simulink model "HandlerSOMANET"  (R2016b)
settings: Solver=VariableStepAuto  StartTime=0.0  StopTime=10.0  RelTol=1e-3
settings Model: DataDictionary=ModelDictionary.sldd  Creator=Nathan  LastModifiedBy=Nathan

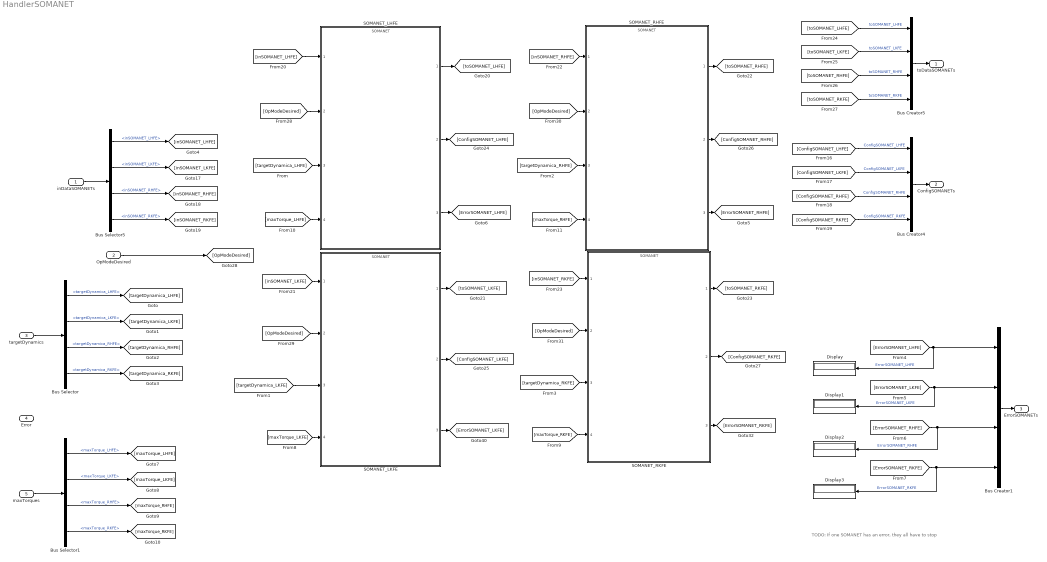
== system HandlerSOMANET ==
  note: TODO: If one SOMANET has an error, they all have to stop
  inDataSOMANETs : Inport  OutDataTypeStr=Bus: inDataSOMANETs  BusOutputAsStruct=on
  OpModeDesired : Inport  Port=2
  targetDynamics : Inport  Port=3  OutDataTypeStr=Bus: targetDynamics  BusOutputAsStruct=on
  Error : Inport  Port=4  BusOutputAsStruct=on
  maxTorques : Inport  Port=5  OutDataTypeStr=Bus: maxTorques  BusOutputAsStruct=on
  Bus Creator1 : BusCreator  Inputs=4  OutDataTypeStr=Bus: toSafetySOMANETs  NonVirtualBus=on
  Bus Creator4 : BusCreator  Inputs=4  OutDataTypeStr=Bus: ConfigSOMANETs  NonVirtualBus=on
  Bus Creator5 : BusCreator  Inputs=4
  Bus Selector : BusSelector  OutputSignals=targetDynamica_LHFE,targetDynamica_LKFE,targetDynamica_RHFE,targetDynamica_RKFE
  Bus Selector1 : BusSelector  OutputSignals=maxTorque_LHFE,maxTorque_LKFE,maxTorque_RHFE,maxTorque_RKFE
  Bus Selector5 : BusSelector  OutputSignals=inSOMANET_LHFE,inSOMANET_LKFE,inSOMANET_RHFE,inSOMANET_RKFE
  Display{,1..3} (4 alike) : Display
  SOMANET_LHFE : ModelReference  ModelNameDialog=SOMANET.slx  SimulationMode=Normal  ModelReferenceVersion=1.37
  SOMANET_LKFE : ModelReference  ModelNameDialog=SOMANET.slx  SimulationMode=Normal  ModelReferenceVersion=1.37
  SOMANET_RHFE : ModelReference  ModelNameDialog=SOMANET.slx  SimulationMode=Normal  ModelReferenceVersion=1.37
  SOMANET_RKFE : ModelReference  ModelNameDialog=SOMANET.slx  SimulationMode=Normal  ModelReferenceVersion=1.37
  toDataSOMANETs : Outport  OutDataTypeStr=Bus: toDataSOMANETs  BusOutputAsStruct=on
  ConfigSOMANETs : Outport  Port=2  OutDataTypeStr=Bus: ConfigSOMANETs  BusOutputAsStruct=on
  ErrorSOMANETs : Outport  Port=3
  wires:
  Bus Creator4/1 -> ConfigSOMANETs/1
  [ConfigSOMANET_LHFE] -> Bus Creator4/1  "ConfigSOMANET_LHFE"
  [ConfigSOMANET_LKFE] -> Bus Creator4/2  "ConfigSOMANET_LKFE"
  [ConfigSOMANET_RHFE] -> Bus Creator4/3  "ConfigSOMANET_RHFE"
  [ConfigSOMANET_RKFE] -> Bus Creator4/4  "ConfigSOMANET_RKFE"
  inDataSOMANETs/1 -> Bus Selector5/1
  Bus Selector5/4 -> [inSOMANET_RKFE]  "<inSOMANET_RKFE>"
  Bus Selector5/3 -> [inSOMANET_RHFE]  "<inSOMANET_RHFE>"
  Bus Selector5/2 -> [inSOMANET_LKFE]  "<inSOMANET_LKFE>"
  Bus Selector5/1 -> [inSOMANET_LHFE]  "<inSOMANET_LHFE>"
  [inSOMANET_LHFE] -> SOMANET_LHFE/1
  [inSOMANET_LKFE] -> SOMANET_LKFE/1
  [inSOMANET_RHFE] -> SOMANET_RHFE/1
  Bus Creator5/1 -> toDataSOMANETs/1
  [toSOMANET_LHFE] -> Bus Creator5/1  "toSOMANET_LHFE"
  [toSOMANET_LKFE] -> Bus Creator5/2  "toSOMANET_LKFE"
  [toSOMANET_RKFE] -> Bus Creator5/4  "toSOMANET_RKFE"
  [toSOMANET_RHFE] -> Bus Creator5/3  "toSOMANET_RHFE"
  SOMANET_LHFE/1 -> [toSOMANET_LHFE]
  SOMANET_LKFE/1 -> [toSOMANET_LKFE]
  SOMANET_RHFE/1 -> [toSOMANET_RHFE]
  SOMANET_RKFE/1 -> [toSOMANET_RKFE]
  SOMANET_LHFE/2 -> [ConfigSOMANET_LHFE]
  SOMANET_LKFE/2 -> [ConfigSOMANET_LKFE]
  SOMANET_RHFE/2 -> [ConfigSOMANET_RHFE]
  SOMANET_RKFE/2 -> [ConfigSOMANET_RKFE]
  OpModeDesired/1 -> [OpModeDesired]
  [OpModeDesired] -> SOMANET_LHFE/2
  [OpModeDesired] -> SOMANET_RHFE/2
  [inSOMANET_RKFE] -> SOMANET_RKFE/1
  [OpModeDesired] -> SOMANET_RKFE/2
  [OpModeDesired] -> SOMANET_LKFE/2
  targetDynamics/1 -> Bus Selector/1
  Bus Selector/1 -> [targetDynamica_LHFE]  "<targetDynamica_LHFE>"
  Bus Selector/2 -> [targetDynamica_LKFE]  "<targetDynamica_LKFE>"
  Bus Selector/3 -> [targetDynamica_RHFE]  "<targetDynamica_RHFE>"
  Bus Selector/4 -> [targetDynamica_RKFE]  "<targetDynamica_RKFE>"
  [targetDynamica_LHFE] -> SOMANET_LHFE/3
  [targetDynamica_LKFE] -> SOMANET_LKFE/3
  [targetDynamica_RHFE] -> SOMANET_RHFE/3
  [targetDynamica_RKFE] -> SOMANET_RKFE/3
  Bus Creator1/1 -> ErrorSOMANETs/1
  SOMANET_LHFE/3 -> [ErrorSOMANET_LHFE]
  SOMANET_RHFE/3 -> [ErrorSOMANET_RHFE]
  SOMANET_LKFE/3 -> [ErrorSOMANET_LKFE]
  SOMANET_RKFE/3 -> [ErrorSOMANET_RKFE]
  [ErrorSOMANET_LHFE] -> Display/1, Bus Creator1/1  "ErrorSOMANET_LHFE"
  [ErrorSOMANET_LKFE] -> Display1/1, Bus Creator1/2  "ErrorSOMANET_LKFE"
  [ErrorSOMANET_RHFE] -> Display2/1, Bus Creator1/3  "ErrorSOMANET_RHFE"
  [ErrorSOMANET_RKFE] -> Display3/1, Bus Creator1/4  "ErrorSOMANET_RKFE"
  maxTorques/1 -> Bus Selector1/1
  Bus Selector1/1 -> [maxTorque_LHFE]  "<maxTorque_LHFE>"
  Bus Selector1/2 -> [maxTorque_LKFE]  "<maxTorque_LKFE>"
  Bus Selector1/3 -> [maxTorque_RHFE]  "<maxTorque_RHFE>"
  Bus Selector1/4 -> [maxTorque_RKFE]  "<maxTorque_RKFE>"
  [maxTorque_LKFE] -> SOMANET_LKFE/4
  [maxTorque_RKFE] -> SOMANET_RKFE/4
  [maxTorque_LHFE] -> SOMANET_LHFE/4
  [maxTorque_RHFE] -> SOMANET_RHFE/4
